simulink model "sgMdl_IO323_AnalogLoopback_Triggered"  (R2024b)
settings: Solver=FixedStepAuto  StartTime=0.0  StopTime=inf  RelTol=1e-3
undefined symbols (not defined in the file): Pull, pull, up
libraries: speedgoatlib_fpga_dio x2, speedgoatlib_fpga_analog_io x2, simulink x1, speedgoatlib_fpga x1
Description:
  | IO323 - Analog Loopback External Triggered
settings Model: ModifiedByFormat=Speedgoat  SimulationMode=external  ExtModeTrigDuration=100000  Creator=Speedgoat  LastModifiedBy=Speedgoat
settings SolverCC: ConcurrentTasks=on  PositivePriorityOrder=on
settings DataIOCC: SaveFormat=StructureWithTime
settings OptimizationCC: BlockReduction=off  OptimizeBlockIOStorage=off  BufferReuse=off  ReuseModelBlockBuffer=off
settings DebuggingCC: UnderspecifiedInitializationDetection=Classic  MergeDetectMultiDrivingBlocksExec=none  TasksWithSamePriorityMsg=none
settings HardwareCC: ProdBitPerLong=64  ProdLongLongMode=on  ProdHWDeviceType=Intel->x86-64 (Linux 64)
settings ModelReferenceCC: EnableRefExpFcnMdlSchedulingChecks=on  PropagateSignalLabelsOutOfModel=off
settings RTWCC: Description=Speedgoat Real-Time Target Machine  SystemTargetFile=speedgoat.tlc  TemplateMakefile=slrealtime_default_tmf  PostCodeGenCommand=sg.model.build.makeCfg(bdroot, buildInfo);  Toolchain=Simulink Real-Time Toolchain  BuildConfiguration=Faster Runs  TargetLang=C++  GPUComputeCapability=3.5
settings SimulinkRealTimeTargetCC: SubcomponentCodeInterfacePackaging=Reusable function  InstructionSetFMA=off  LogToMDFFile=off  SLRTFileLogMaxRuns=10
settings ConfigComp: CovBoundaryAbsTol=1.0e-5

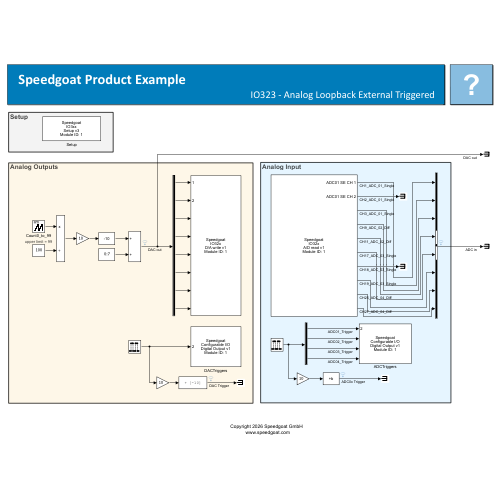
[thumbnail: Simulink's stored preview of the top-level diagram]
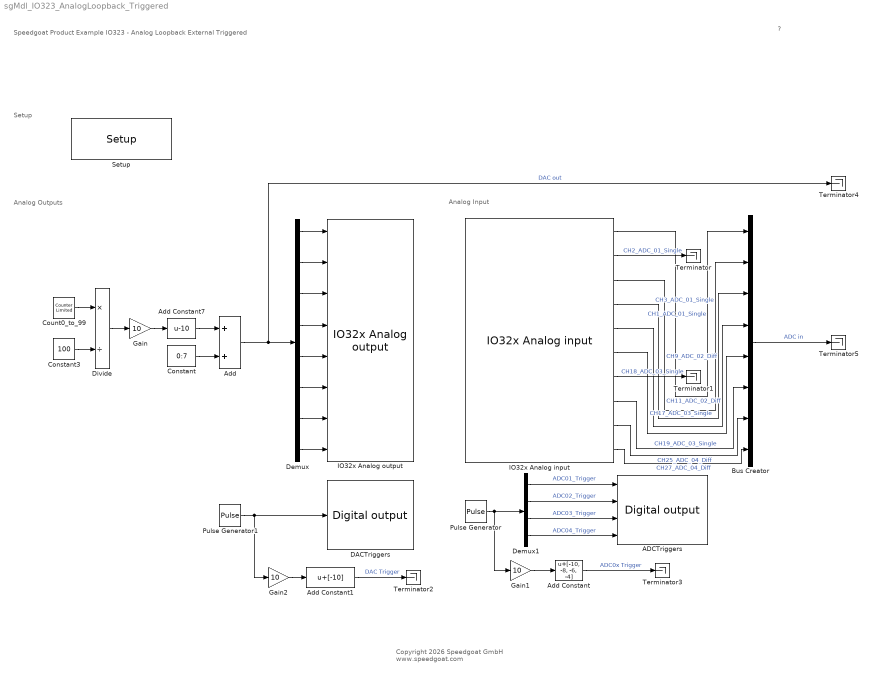
== system sgMdl_IO323_AnalogLoopback_Triggered ==
  note: Analog Outputs
  note: Analog Input
  note: Setup
  note: Speedgoat Product Example
      | IO323 - Analog Loopback External Triggered
  note: ?
  note: Copyright 2026 Speedgoat GmbH
      |  www.speedgoat.com
  ADCTriggers : speedgoatlib_fpga_dio/Digital output  id=1  chan=20:23  init=[0]  reset=[0]  ts=1e-3  vectorizeInput=off
      settings: SourceProductName=Simulink Real-Time: Speedgoat I/O Blockset
  Add : Sum
  Add Constant : Bias  Bias=[-10, -8, -6, -4]  SaturateOnIntegerOverflow=off
  Add Constant1 : Bias  Bias=[-10]  SaturateOnIntegerOverflow=off
  Add Constant7 : Bias  Bias=-10  SaturateOnIntegerOverflow=off
  Bus Creator : BusCreator  Inputs=8
  Constant : Constant  Value=0:7  SampleTime=-1
  Constant3 : Constant  Value=100  SampleTime=-1
  Count0_to_99 : simulink/Sources/Counter Limited  uplimit=99  tsamp=-1
      settings: AttributesFormatString=upper limit = %<uplimit>
  DACTriggers : speedgoatlib_fpga_dio/Digital output  id=1  chan=24  init=[0]  reset=[0]  ts=1e-3  vectorizeInput=off
      settings: SourceProductName=Simulink Real-Time: Speedgoat I/O Blockset
  Demux : Demux  Outputs=8
  Demux1 : Demux
  Divide : Product  Inputs=*/
  Gain : Gain  Gain=10
  Gain1 : Gain  Gain=10
  Gain2 : Gain  Gain=10
  IO32x Analog input : speedgoatlib_fpga_analog_io/IO32x/IO32x Analog input  Priority=1  id=1  ts=10e-3  ADC1_chan=[1 2 3]  ADC1_range=+-10.24 V  ADC1_diff=Single-ended  ADC1_Trigger=Target  ADC1_Seq=on  ADC2_chan=[1 2]  ADC2_range=+-10.24 V  ADC2_diff=Differential  ADC2_Trigger=Target  ADC2_Seq=on  ADC3_chan=[1 2 3]  ADC3_range=+-10.24 V  ADC3_diff=Single-ended  ADC3_Trigger=Target  ADC3_Seq=on  ADC4_chan=[1 2]  ADC4_range=+-10.24 V  ADC4_diff=Differential  ADC4_Trigger=Target  ADC4_Seq=on
      settings: SourceProductName=Simulink Real-Time: Speedgoat I/O Blockset
  IO32x Analog output : speedgoatlib_fpga_analog_io/IO32x/IO32x Analog output  Priority=2  id=1  chan=[1:8]  trigger=Target  initVal=[-10 -9 -8 -7 -6 -5 -4 -3]  resetVal=[1 0 1 0 1 0 1 0]  ts=10e-3  pciSlot=-1  board=IO323
      settings: SourceProductName=Simulink Real-Time: Speedgoat I/O Blockset
  Pulse Generator : DiscretePulseGenerator  Period=120  PulseWidth=[120 1 1 1]  PhaseDelay=[0 6 46 86]  SampleTime=-1
  Pulse Generator1 : DiscretePulseGenerator  Period=40  PhaseDelay=4  SampleTime=-1
  Setup : speedgoatlib_fpga/Setup/Setup  board=IO323  id=1  pciSlot=-1  device_id=1  bitstreamFilePath=[]  bitstreamFile=speedgoat_IO323_CI_02613_test  fpgaFreq=75 MHz  enableDma=off  rearEnb_1=off  rearIO_1=None  rearEnb_2=off  rearIO_2=None  ProgSpiFlash=off  ProgBPIFlash=off  useFpgaDmaController=off  dmaTrigDropdown=Model Step  dmaTrigSelect=0  dmaStopOnOverload=on  dmaModeSequential=on  dmaModeParallel=off  PullRPort15=pull-up 3.3V  PullRPort31=pull-up 3.3V  PullRPort47=pull-up 3.3V  PullRPort63=pull-up 3.3V  diffLineTermination_1=on  diffLineTermination_2=on  diffLineTermination_3=on  diffLineTermination_4=on  diffLineTermination_5=on  diffLineTermination_6=on  diffLineTermination_7=on  diffLineTermination_8=on  diffLineTermination_9=on  diffLineTermination_10=on  diffLineTermination_11=on  diffLineTermination_12=on  diffLineTermination_13=on  diffLineTermination_14=on  diffLineTermination_15=on  diffLineTermination_16=on  diffLineTermination_17=on  diffLineTermination_18=on  diffLineTermination_19=on  diffLineTermination_20=on  diffLineTermination_21=on  diffLineTermination_22=on  diffLineTermination_23=on  diffLineTermination_24=on  diffLineTermination_25=on  diffLineTermination_26=on  diffLineTermination_27=on  diffLineTermination_28=on  diffLineTermination_29=on  diffLineTermination_30=on  diffLineTermination_31=on  diffLineTermination_32=on  ioVoltageDropDown1=3.3V  pullResistorDropDown1_1=Pull-up  pullResistorDropDown1_2=Pull-up  pullResistorDropDown1_3=Pull-up  pullResistorDropDown1_4=Pull-up  pullResistorDropDown1_5=Pull-up  pullResistorDropDown1_6=Pull-up  pullResistorDropDown1_7=Pull-up  pullResistorDropDown1_8=Pull-up  ttlIsImplementedCheckBox1=off  pullResistorDropDown2=Pull-up  ioVoltageDropDown2=3.3V  ttlIsImplementedCheckBox2=off  pullResistorDropDown3=Pull-up  ioVoltageDropDown3=3.3V  ttlIsImplementedCheckBox3=off  pullResistorDropDown4=Pull-up  ioVoltageDropDown4=3.3V  ttlIsImplementedCheckBox4=off  pullResistorDropDown5=Pull-up  ioVoltageDropDown5=3.3V  ttlIsImplementedCheckBox5=off  pullResistorDropDown6=Pull-up  ioVoltageDropDown6=3.3V  ttlIsImplementedCheckBox6=off  pullResistorDropDown7=Pull-up  ioVoltageDropDown7=3.3V  ttlIsImplementedCheckBox7=off  pullResistorDropDown8=Pull-up  ioVoltageDropDown8=3.3V  ttlIsImplementedCheckBox8=off  terminationCheckBox1=off  terminationCheckBox2=off  terminationCheckBox3=off  terminationCheckBox4=off  diffIsImplementedCheckBox1=off  terminationCheckBox5=off  terminationCheckBox6=off  terminationCheckBox7=off  terminationCheckBox8=off  diffIsImplementedCheckBox2=off  terminationCheckBox9=off  terminationCheckBox10=off  terminationCheckBox11=off  terminationCheckBox12=off  diffIsImplementedCheckBox3=off  terminationCheckBox13=off  terminationCheckBox14=off  terminationCheckBox15=off  terminationCheckBox16=off  diffIsImplementedCheckBox4=off  terminationCheckBox17=off  terminationCheckBox18=off  terminationCheckBox19=off  terminationCheckBox20=off  diffIsImplementedCheckBox5=off  terminationCheckBox21=off  terminationCheckBox22=off  terminationCheckBox23=off  terminationCheckBox24=off  diffIsImplementedCheckBox6=off  terminationCheckBox25=off  terminationCheckBox26=off  terminationCheckBox27=off  terminationCheckBox28=off  diffIsImplementedCheckBox7=off  terminationCheckBox29=off  terminationCheckBox30=off  terminationCheckBox31=off  terminationCheckBox32=off  diffIsImplementedCheckBox8=off  PullRPort0_1=pull-up  VioPort0_1=3.3V  PullRPort1_1=pull-up  VioPort1_1=3.3V  PullRPort2_1=pull-up  VioPort2_1=3.3V  PullRPort3_1=pull-up  VioPort3_1=3.3V  PullRPort4_1=pull-up  VioPort4_1=3.3V  PullRPort5_1=pull-up  VioPort5_1=3.3V  PullRPort6_1=pull-up  VioPort6_1=3.3V  diffLineTermination_rear1_1=on  diffLineTermination_rear1_2=on  diffLineTermination_rear1_3=on  diffLineTermination_rear1_4=on  diffLineTermination_rear1_5=on  diffLineTermination_rear1_6=on  diffLineTermination_rear1_7=on  diffLineTermination_rear1_8=on  PullRPort0_2=pull-up  VioPort0_2=3.3V  PullRPort1_2=pull-up  VioPort1_2=3.3V  PullRPort2_2=pull-up  VioPort2_2=3.3V  PullRPort3_2=pull-up  VioPort3_2=3.3V  PullRPort4_2=pull-up  VioPort4_2=3.3V  PullRPort5_2=pull-up  VioPort5_2=3.3V  PullRPort6_2=pull-up  VioPort6_2=3.3V  diffLineTermination_rear2_1=on  diffLineTermination_rear2_2=on  diffLineTermination_rear2_3=on  diffLineTermination_rear2_4=on  diffLineTermination_rear2_5=on  diffLineTermination_rear2_6=on  diffLineTermination_rear2_7=on  diffLineTermination_rear2_8=on
      settings: SourceProductName=Simulink Real-Time: Speedgoat I/O Blockset
  Terminator{,1..5} (6 alike) : Terminator
  wires:
  Divide/1 -> Gain/1
  Constant3/1 -> Divide/2
  Count0_to_99/1 -> Divide/1
  Gain/1 -> Add Constant7/1
  Add Constant7/1 -> Add/1
  Demux/3 -> IO32x Analog output/3
  Demux/5 -> IO32x Analog output/5
  Demux/4 -> IO32x Analog output/4
  Demux/8 -> IO32x Analog output/8
  Demux/6 -> IO32x Analog output/6
  Demux/7 -> IO32x Analog output/7
  Demux/1 -> IO32x Analog output/1
  Demux/2 -> IO32x Analog output/2
  Constant/1 -> Add/2
  Add/1 -> Terminator4/1, Demux/1  "DAC out"
  Demux1/2 -> ADCTriggers/2  "ADC02_Trigger"
  Demux1/3 -> ADCTriggers/3  "ADC03_Trigger"
  Demux1/1 -> ADCTriggers/1  "ADC01_Trigger"
  Demux1/4 -> ADCTriggers/4  "ADC04_Trigger"
  Pulse Generator/1 -> Gain1/1, Demux1/1
  Pulse Generator1/1 -> Gain2/1, DACTriggers/1
  Gain1/1 -> Add Constant/1
  Gain2/1 -> Add Constant1/1
  Add Constant1/1 -> Terminator2/1  "DAC Trigger"
  Add Constant/1 -> Terminator3/1  "ADC0x Trigger"
  Bus Creator/1 -> Terminator5/1  "ADC in"
  IO32x Analog input/2 -> Terminator/1  "CH2_ADC_01_Single"
  IO32x Analog input/5 -> Bus Creator/4  "CH11_ADC_02_Diff"
  IO32x Analog input/1 -> Bus Creator/1  "CH1_ADC_01_Single"
  IO32x Analog input/4 -> Bus Creator/3  "CH9_ADC_02_Diff"
  IO32x Analog input/6 -> Bus Creator/5  "CH17_ADC_03_Single"
  IO32x Analog input/8 -> Bus Creator/6  "CH19_ADC_03_Single"
  IO32x Analog input/9 -> Bus Creator/7  "CH25_ADC_04_Diff"
  IO32x Analog input/3 -> Bus Creator/2  "CH3_ADC_01_Single"
  IO32x Analog input/10 -> Bus Creator/8  "CH27_ADC_04_Diff"
  IO32x Analog input/7 -> Terminator1/1  "CH18_ADC_03_Single"
